simulink model "SMC"  (Simulink 7.5)
settings: Solver=ode45  StartTime=0.0  StopTime=10.0  MaxStep=0.02  RelTol=1e-3
settings Model: Creator=Administrador  LastModifiedBy=jorgesofrony
settings OptimizationCC: InitFltsAndDblsToZero=on
settings DebuggingCC: StrictBusMsg=Warning

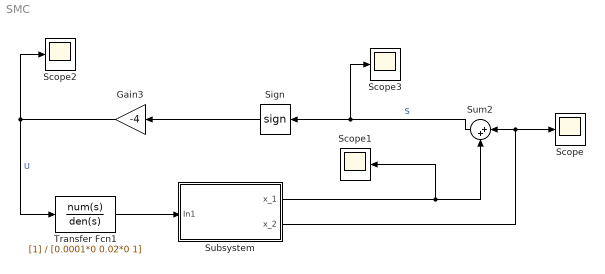
== system SMC ==
  Gain3 : Gain  Gain=-4  ParameterDataType=sfix(16)  ParameterScaling=2^0  OutDataType=sfix(16)  OutScaling=2^0
  Scope{,1..3} (4 alike) : Scope
      Scope settings: YMin=-1.25e-005  YMax=1e-005
      Scope1 settings: YMin=-1.6165e-005  YMax=-1.61e-005
      Scope2 settings: YMin=-100  YMax=100  SaveName=ScopeData2
      Scope3 settings: YMin=-1.25e-005  YMax=1e-005  SaveName=ScopeData4
  Sign : Signum  ZeroCross=off
  Subsystem : Subsystem
  Sum2 : Sum  Inputs=|++  OutDataType=sfix(16)  OutScaling=2^0
  Transfer Fcn1 : TransferFcn  Denominator=[0.0001*0 0.02*0 1]
  wires:
  Sum2/1 -> Scope3/1, Sign/1  "S"
  Sign/1 -> Gain3/1
  Gain3/1 -> Scope2/1, Transfer Fcn1/1  "U"
  Subsystem/1(x_1) -> Sum2/2, Scope1/1
  Subsystem/2(x_2) -> Sum2/1, Scope/1
  Transfer Fcn1/1 -> Subsystem/1(In1)

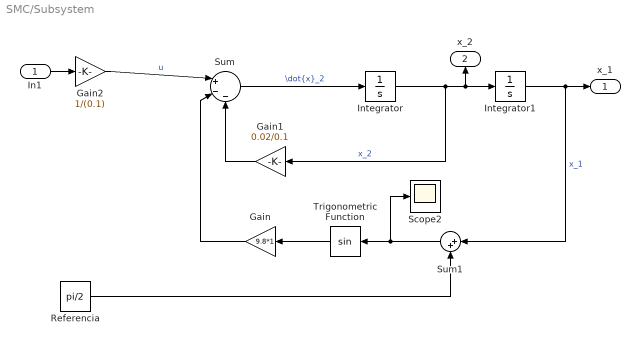
== system SMC/Subsystem ==
  In1 : Inport
  Gain : Gain  Gain=9.8*1  ParameterDataType=sfix(16)  ParameterScaling=2^0  OutDataType=sfix(16)  OutScaling=2^0
  Gain1 : Gain  Gain=0.02/0.1  ParameterDataType=sfix(16)  ParameterScaling=2^0  OutDataType=sfix(16)  OutScaling=2^0
  Gain2 : Gain  Gain=1/(0.1)  ParameterDataType=sfix(16)  ParameterScaling=2^0  OutDataType=sfix(16)  OutScaling=2^0
  Integrator : Integrator
  Integrator1 : Integrator  InitialCondition=-pi/2
  Referencia : Constant  Value=pi/2  OutDataType=sfix(16)  OutScaling=2^0
  Scope2 : Scope
      settings: YMin=1.57078  YMax=1.57079  SaveName=ScopeData3
  Sum : Sum  Inputs=|+--  OutDataType=sfix(16)  OutScaling=2^0
  Sum1 : Sum  Inputs=|++  OutDataType=sfix(16)  OutScaling=2^0
  Trigonometric Function : Trigonometry
  x_1 : Outport
  x_2 : Outport  Port=2
  wires:
  Referencia/1 -> Sum1/2
  Gain2/1 -> Sum/1  "u"
  In1/1 -> Gain2/1
  Sum/1 -> Integrator/1  "\\dot{x}_2"
  Gain/1 -> Sum/2
  Gain1/1 -> Sum/3
  Trigonometric Function/1 -> Gain/1
  Sum1/1 -> Trigonometric Function/1, Scope2/1
  Integrator1/1 -> Sum1/1, x_1/1  "x_1"
  Integrator/1 -> Gain1/1, Integrator1/1, x_2/1  "x_2"
